simulink model "ex1"  (R2018a)
settings: Solver=VariableStepAuto  StartTime=0.0  StopTime=10.0  RelTol=1e-3
settings Model: Creator=DELL  LastModifiedBy=DELL

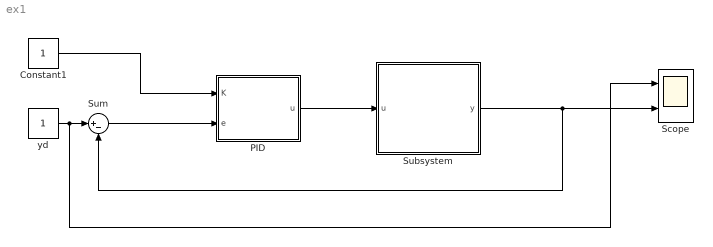
== system ex1 ==
  Constant1 : Constant
  PID : Subsystem
  Scope : Scope  NumInputPorts=2
  Subsystem : Subsystem  mask{m=1, l=0.6, b=0.1, g=9.81}
      mask prompts: m "khoi luong con lac"; l "chieu dai con lac"; b "he so ma sat"; g "gia toc"
  Sum : Sum  Inputs=|+-
  yd : Constant
  wires:
  PID/1(u) -> Subsystem/1(u)
  Sum/1 -> PID/2(e)
  yd/1 -> Scope/1, Sum/1
  Constant1/1 -> PID/1(K)
  Subsystem/1(y) -> Scope/2, Sum/2

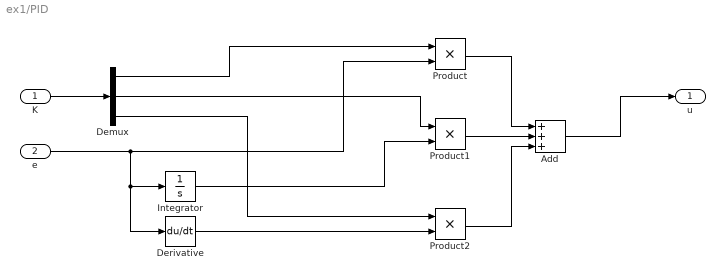
== system ex1/PID ==
  K : Inport
  e : Inport  Port=2
  Add : Sum  Inputs=+++
  Demux : Demux  Outputs=3
  Derivative : Derivative
  Integrator : Integrator
  Product : Product
  Product1 : Product
  Product2 : Product
  u : Outport
  wires:
  K/1 -> Demux/1
  Demux/1 -> Product/1
  e/1 -> Integrator/1, Derivative/1, Product/2
  Integrator/1 -> Product1/2
  Demux/2 -> Product1/1
  Demux/3 -> Product2/1
  Derivative/1 -> Product2/2
  Product/1 -> Add/1
  Product1/1 -> Add/2
  Product2/1 -> Add/3
  Add/1 -> u/1

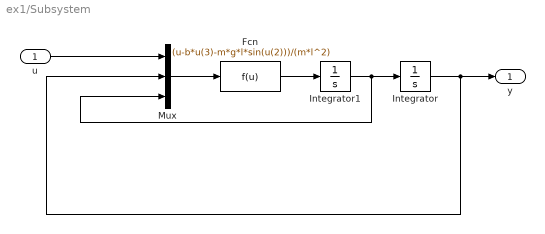
== system ex1/Subsystem ==
  u : Inport
  Fcn : Fcn  Expr=(u-b*u(3)-m*g*l*sin(u(2)))/(m*l^2)
  Integrator : Integrator
  Integrator1 : Integrator
  Mux : Mux  Inputs=3
  y : Outport
  wires:
  Integrator/1 -> Mux/2, y/1
  Fcn/1 -> Integrator1/1
  Mux/1 -> Fcn/1
  u/1 -> Mux/1
  Integrator1/1 -> Mux/3, Integrator/1
